simulink model "RLC_square_wave"  (R2018b)
settings: Solver=VariableStepAuto  StartTime=0.0  StopTime=0.01  RelTol=1e-3
model workspace (MATLAB code in the model file):
  | C = 0.22e-6; % F
  | R = 180; % Ohm
  | L =50e-3; %H
settings Model: Creator=kjartan  LastModifiedBy=kjartan

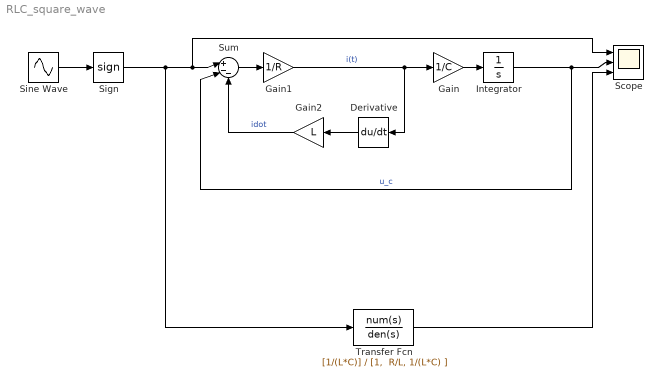
== system RLC_square_wave ==
  Derivative : Derivative  CoefficientInTFapproximation=0.01
  Gain : Gain  Gain=1/C
  Gain1 : Gain  Gain=1/R
  Gain2 : Gain  Gain=L
  Integrator : Integrator
  Scope : Scope  NumInputPorts=3
  Sign : Signum
  Sine Wave : Sin  Frequency=2*pi*200  SampleTime=0
  Sum : Sum  Inputs=|+--
  Transfer Fcn : TransferFcn  Numerator=[1/(L*C)]  Denominator="[1,  R/L, 1/(L*C) ]"
  wires:
  Integrator/1 -> Sum/2, Scope/2  "u_c"
  Gain/1 -> Integrator/1
  Gain1/1 -> Derivative/1, Gain/1  "i(t)"
  Sign/1 -> Transfer Fcn/1, Scope/1, Sum/1
  Sum/1 -> Gain1/1
  Sine Wave/1 -> Sign/1
  Derivative/1 -> Gain2/1
  Gain2/1 -> Sum/3  "idot"
  Transfer Fcn/1 -> Scope/3
